simulink model "Demo1_P2C4"  (R2025b)
settings: Solver=VariableStepAuto  StartTime=0.0  StopTime=10.0  RelTol=1e-3
undefined symbols (not defined in the file): k
settings Model: Creator=abadirwahba  LastModifiedBy=abadirwahba

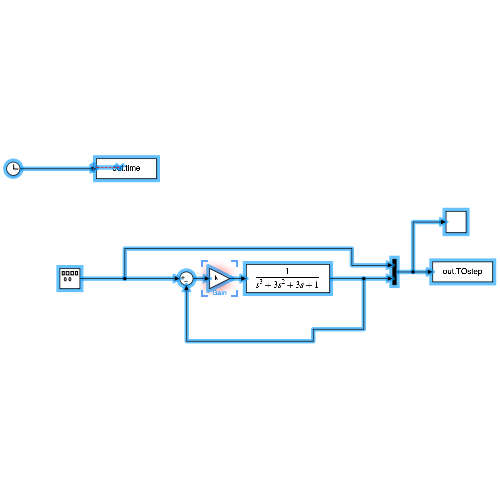
[thumbnail: Simulink's stored preview of the top-level diagram]
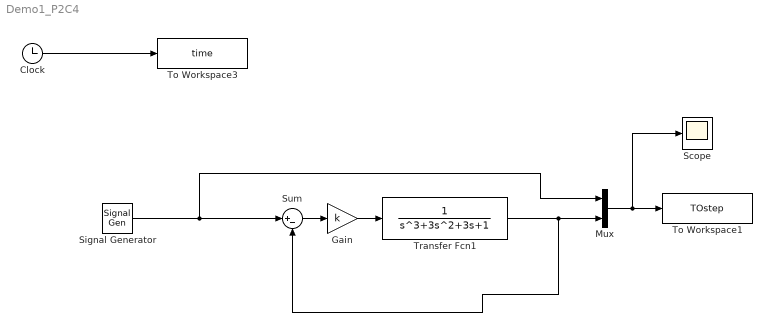
== system Demo1_P2C4 ==
  Clock : Clock
  Gain : Gain  Gain=k
  Mux : Mux  Inputs=2
  Scope : Scope
      settings: ActiveDisplayYMinimum=-98143.816559128623  ActiveDisplayYMaximum=90132.524799049163
  Signal Generator : SignalGenerator  WaveForm=square  Frequency=0.01
  Sum : Sum  Inputs=|+-
  To Workspace1 : ToWorkspace  VariableName=TOstep  SampleTime=-1
  To Workspace3 : ToWorkspace  VariableName=time  SampleTime=-1
  Transfer Fcn1 : TransferFcn  Denominator=[1 3 3 1]
  wires:
  Clock/1 -> To Workspace3/1
  Sum/1 -> Gain/1
  Signal Generator/1 -> Sum/1, Mux/1
  Transfer Fcn1/1 -> Sum/2, Mux/2
  ? -> ?
  Mux/1 -> Scope/1, To Workspace1/1
  Gain/1 -> Transfer Fcn1/1
